simulink model "HalfBridge"  (R2024a)
settings: Solver=VariableStepAuto  StartTime=0.0  StopTime=2e-3  FixedStep=2e-7  RelTol=1e-3
libraries: spsVoltageMeasurementLib x5, spsSeriesRLCBranchLib x4, spsGroundLib x3, spsDiodeLib x2, spsCurrentMeasurementLib x2, spsMosfetLib x2, spsDCVoltageSourceLib x1, spsMutualInductanceLib x1, sps_lib x1
settings Model: Creator=shouyu  LastModifiedBy=shouyu

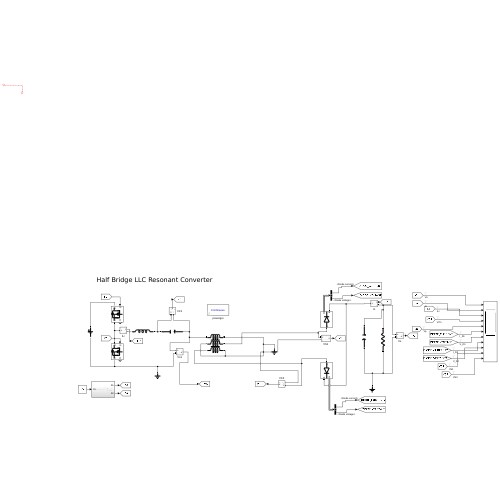
[thumbnail: Simulink's stored preview of the top-level diagram]
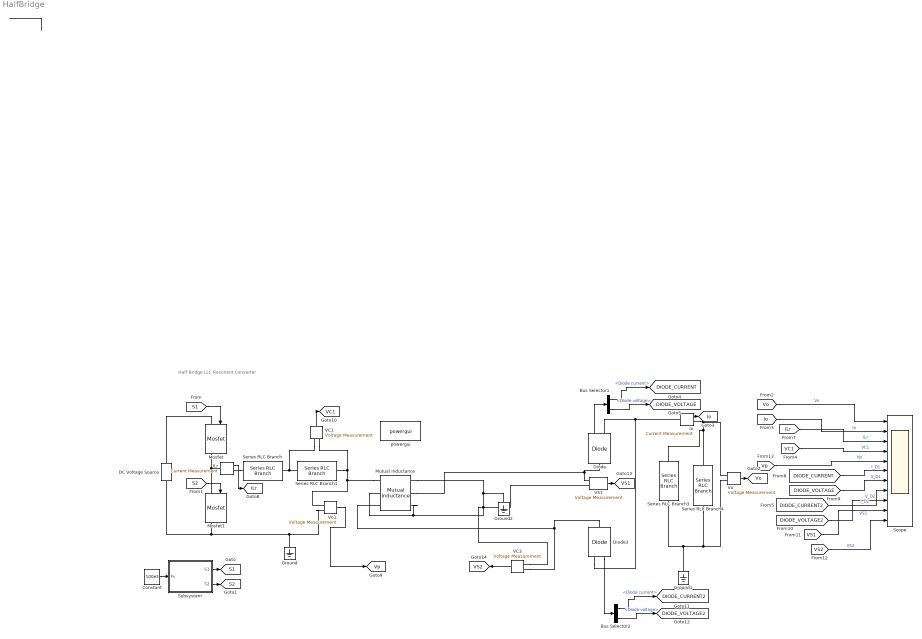
== system HalfBridge ==
  note: Half Bridge LLC Resonant Converter
  Bus Selector1 : BusSelector  OutputSignals=Diode current,Diode voltage
  Bus Selector2 : BusSelector  OutputSignals=Diode current,Diode voltage
  Constant : Constant  Value=100e3
  DC Voltage Source : spsDCVoltageSourceLib/DC Voltage Source  Amplitude=400  Measurements=None
  Diode : spsDiodeLib/Diode  Ron=0.001  Lon=0  Vf=0  IC=0  UseSnubber=0  Rs=0  Cs=0  Measurements=on
  Diode3 : spsDiodeLib/Diode  Ron=0.001  Lon=0  Vf=0  IC=0  UseSnubber=0  Rs=0  Cs=0  Measurements=on
  Ground : spsGroundLib/Ground  LConnTagsString=a
  Ground1 : spsGroundLib/Ground  LConnTagsString=a
  Ground2 : spsGroundLib/Ground  LConnTagsString=a
  ILr : spsCurrentMeasurementLib/Current Measurement  PhasorSimulation=off  OutputType=Complex  PSBequivalent=0
  Io : spsCurrentMeasurementLib/Current Measurement  PhasorSimulation=off  OutputType=Complex  PSBequivalent=0
  Mosfet : spsMosfetLib/Mosfet  Ron=0.1  Lon=0  Rd=0  Vfd=0  IC=0  Rs=0  Cs=0  Measurements=on
  Mosfet1 : spsMosfetLib/Mosfet  Ron=0.1  Lon=0  Rd=0  Vfd=0  IC=0  Rs=0  Cs=0  Measurements=on
  Mutual Inductance : spsMutualInductanceLib/Mutual Inductance  LConnTagsString=a|b|c  RConnTagsString=A|B|C  TypeOfMutual=Generalized mutual inductance  NumberOfWindings=3  SelfImpedance1=[1.1 1.1e-03]  SelfImpedance2=[ 1.1 1.1e-03]  ThreeWindings=on  SelfImpedance3=[ 1.1 1.1e-03]  MutualImpedance=[1.0 1.0e-03]  InductanceMatrix=[280e-6 1.6298e-5 1.6298e-5; 1.6298e-5 968e-9 9.5832e-7; 1.6298e-5 9.5832e-7 968e-9]  ResistanceMatrix=[0 0 0; 0 0 0; 0 0 0]  Measurements=None
      settings: LibrarySourceBlock=sps_lib/Passives/Mutual Inductance
  Scope : Scope  NumInputPorts=11
  Series RLC Branch : spsSeriesRLCBranchLib/Series RLC Branch  LConnTagsString=__new0  RConnTagsString=__new0  BranchType=L  Resistance=0.01  Inductance=60e-6  SetiL0=off  InitialCurrent=0  Capacitance=1e-6  Setx0=off  InitialVoltage=0  Measurements=None
  Series RLC Branch1 : spsSeriesRLCBranchLib/Series RLC Branch  LConnTagsString=__new0  RConnTagsString=__new0  BranchType=C  Resistance=1  Inductance=1e-3  SetiL0=off  InitialCurrent=0  Capacitance=24e-9  Setx0=off  InitialVoltage=0  Measurements=None
  Series RLC Branch3 : spsSeriesRLCBranchLib/Series RLC Branch  LConnTagsString=__new0  RConnTagsString=__new0  BranchType=C  Resistance=1  Inductance=1e-3  SetiL0=off  InitialCurrent=0  Capacitance=1000e-6  Setx0=off  InitialVoltage=0  Measurements=None
  Series RLC Branch4 : spsSeriesRLCBranchLib/Series RLC Branch  LConnTagsString=__new0  RConnTagsString=__new0  BranchType=R  Resistance=0.48  Inductance=1e-3  SetiL0=off  InitialCurrent=0  Capacitance=1e-6  Setx0=off  InitialVoltage=0  Measurements=None
  Subsystem : Subsystem
  VC1 : spsVoltageMeasurementLib/Voltage Measurement  PhasorSimulation=off  OutputType=Complex  PSBequivalent=0
  VC3 : spsVoltageMeasurementLib/Voltage Measurement  PhasorSimulation=off  OutputType=Complex  PSBequivalent=0
  VS1 : spsVoltageMeasurementLib/Voltage Measurement  PhasorSimulation=off  OutputType=Complex  PSBequivalent=0
  Vo : spsVoltageMeasurementLib/Voltage Measurement  PhasorSimulation=off  OutputType=Complex  PSBequivalent=0
  Vo1 : spsVoltageMeasurementLib/Voltage Measurement  PhasorSimulation=off  OutputType=Complex  PSBequivalent=0
  powergui : sps_lib/powergui  Priority=1  SimulationMode=Continuous  SampleTime=50e-6  frequency=60  Iterations=50  frequencyindice=0  Pbase=100e6  ErrMax=1e-4  UnitsV=kV  UnitsW=MW  buscounter=0  FunctionMessages=off  echomessages=off  EnableUseOfTLC=off  CurrentSourceSwitches=off  DisableSnubberDevices=off  DisableRonSwitches=off  DisableVfSwitches=off  DisplayEquations=off  AutomaticDiscreteSolvers=off  SolverType=Tustin/Backward Euler (TBE)  Interpol=off  ExternalGateDelay=off  methode=off  Ts=100  x0status=blocks  SPID=on  SwTol=0  HookPort=off  NonlinearTolerance=0  nMaxIteration=15  ContinueOnMaxIteration=off  RestoreLinks=warning  ResistiveCurrentMeasurement=off  Frange=[0:2:500]  Ylog=off  Xlog=on  ShowGrid=off  save=off  variable=ZData  structure=0  ZoomFFT=off  StartTime=0.0  cycles=1  DisplayStyle=1  fundamental=60  FreqAxis=off  MaxFrequency=1000  frequencyindicesteady=1  RmsSteady=1  display=off
  tag scope: DIODE_CURRENT2=global, DIODE_CURRENT=global, DIODE_VOLTAGE2=global, DIODE_VOLTAGE=global, ILr=global, Io=global, S1=global, S2=global, VC1=global, VS1=global, VS2=global, Vo=global, Vp=global
  wires:
  Bus Selector1/1 -> [DIODE_CURRENT]  "<Diode current>"
  Vo/1 -> [Vo]
  Subsystem/1(S1) -> [S1]
  Constant/1 -> Subsystem/1(" Fs")
  [S2] -> Mosfet1/1
  [S1] -> Mosfet/1
  Bus Selector1/2 -> [DIODE_VOLTAGE]  "<Diode voltage>"
  Subsystem/2(S2) -> [S2]
  ILr/1 -> [ILr]
  [Io] -> Scope/2  "Io"
  Diode/1 -> Bus Selector1/1
  [Vo] -> Scope/1  "Vo"
  Io/1 -> [Io]
  Vo1/1 -> [Vp]
  Bus Selector2/2 -> [DIODE_VOLTAGE2]  "<Diode voltage>"
  Bus Selector2/1 -> [DIODE_CURRENT2]  "<Diode current>"
  Diode3/1 -> Bus Selector2/1
  [ILr] -> Scope/3  "ILr"
  [VC1] -> Scope/4  "VC1"
  [DIODE_VOLTAGE] -> Scope/7  "V_D1"
  [DIODE_CURRENT] -> Scope/6  "I_D1"
  VC1/1 -> [VC1]
  VS1/1 -> [VS1]
  VC3/1 -> [VS2]
  [DIODE_CURRENT2] -> Scope/8  "I_D2"
  [DIODE_VOLTAGE2] -> Scope/9  "V_D2"
  [VS1] -> Scope/10  "VS1"
  [VS2] -> Scope/11  "VS2"
  [Vp] -> Scope/5  "Vp"
  connections:
  ?
  Series RLC Branch4/RConn1 -- Ground1/LConn1 -- Series RLC Branch3/RConn1 -- Vo/LConn2
  Io/LConn1 -- Diode3/RConn1 -- Diode/RConn1
  Mosfet1/RConn1 -- Vo1/LConn2 -- Ground/LConn1 -- DC Voltage Source/LConn1
  Mosfet/RConn1 -- Mosfet1/LConn1 -- ILr/LConn1
  Io/RConn1 -- Vo/LConn1 -- Series RLC Branch3/LConn1 -- Series RLC Branch4/LConn1
  DC Voltage Source/RConn1 -- Mosfet/LConn1
  ILr/RConn1 -- Series RLC Branch/LConn1
  Mutual Inductance/LConn1 -- Vo1/LConn1 -- Series RLC Branch1/RConn1 -- VC1/LConn2
  Diode/LConn1 -- Mutual Inductance/RConn2 -- VS1/LConn1
  VC3/LConn1 -- Mutual Inductance/LConn3 -- Diode3/LConn1
  VS1/LConn2 -- VC3/LConn2 -- Mutual Inductance/RConn3 -- Mutual Inductance/LConn2 -- Mutual Inductance/RConn1 -- Ground2/LConn1
  Series RLC Branch1/LConn1 -- VC1/LConn1 -- Series RLC Branch/RConn1

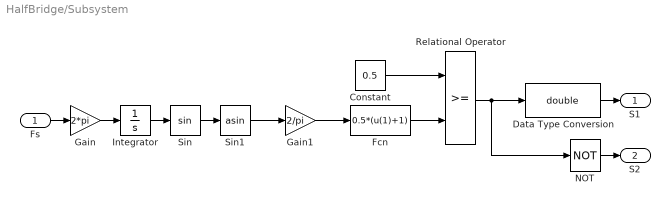
== system HalfBridge/Subsystem ==
  " Fs" : Inport
  Constant : Constant  Value=0.5
  Data Type Conversion : DataTypeConversion  OutDataTypeStr=double  SaturateOnIntegerOverflow=off  RndMeth=Floor
  Fcn : Fcn  Expr=0.5*(u(1)+1)
  Gain : Gain  Gain=2*pi
  Gain1 : Gain  Gain=2/pi
  Integrator : Integrator
  NOT : Logic  Operator=NOT  IconShape=distinctive  AllPortsSameDT=off  OutDataTypeStr=boolean
  Relational Operator : RelationalOperator  OutDataTypeStr=boolean  RndMeth=Simplest  InputSameDT=off
  Sin : Trigonometry
  Sin1 : Trigonometry  Operator=asin
  S1 : Outport  VectorParamsAs1DForOutWhenUnconnected=off
  S2 : Outport  Port=2  VectorParamsAs1DForOutWhenUnconnected=off
  wires:
  Integrator/1 -> Sin/1
  Constant/1 -> Relational Operator/1
  Sin1/1 -> Gain1/1
  Sin/1 -> Sin1/1
  Relational Operator/1 -> NOT/1, Data Type Conversion/1
  Gain/1 -> Integrator/1
  Gain1/1 -> Fcn/1
  Fcn/1 -> Relational Operator/2
  NOT/1 -> S2/1
  " Fs"/1 -> Gain/1
  Data Type Conversion/1 -> S1/1
